simulink model "Yaw_Gearbox_Testrig"  (Simulink 7.9)
settings: Solver=ode23t  StartTime=0.0  StopTime=300  RelTol=1e-3
undefined symbols (not defined in the file): radps2rpm
libraries: fl_lib x9, nesl_utility x3, simulink x1, Yaw_Gearbox_Lib x1
Description:
  | Copyright 2011 MathWorks, Inc.
settings Model: Creator=smiller  LastModifiedBy=smiller
settings DebuggingCC: SolverPrmCheckMsg=none  FcnCallInpInsideContextMsg=Use local settings  StrictBusMsg=Warning
settings GRTTargetCC: CombineOutputUpdateFcns=off  GRTInterface=on

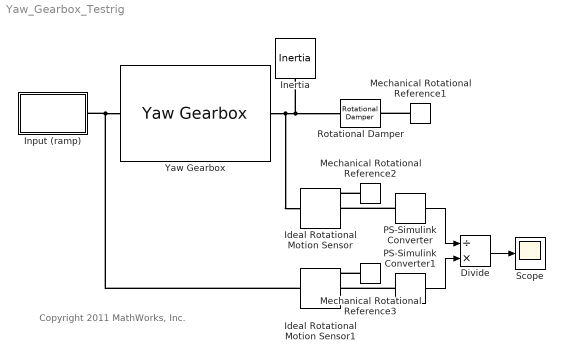
== system Yaw_Gearbox_Testrig ==
  note: Copyright 2011 MathWorks, Inc.
  Divide : Product  Inputs=/*
  Ideal Rotational Motion Sensor : fl_lib/Mechanical/Mechanical Sensors/Ideal Rotational Motion Sensor  offset=0 rad  w_Log=off  t_Log=off  phi_Log=off  LocalVarNames=|w|t|phi  LocalVarDescs=|w|t|phi  LocalVarLogging=[0 0 0]
  Ideal Rotational Motion Sensor1 : fl_lib/Mechanical/Mechanical Sensors/Ideal Rotational Motion Sensor  offset=0 rad  w_Log=off  t_Log=off  phi_Log=off  LocalVarNames=|w|t|phi  LocalVarDescs=|w|t|phi  LocalVarLogging=[0 0 0]
  Inertia : fl_lib/Mechanical/Rotational Elements/Inertia  inertia=1e5 kg*m^2  initial_velocity=0 rad/s  t_Log=off  LocalVarNames=|t  LocalVarDescs=|t  LocalVarLogging=0
  Input (ramp) : Subsystem  mask{start_speed=0, final_speed=14.3004, start_time=3, stop_time=10}
      mask prompts: start_speed "Start speed (rpm)"; final_speed "Final speed (rpm)"; start_time "Ramp start time"; stop_time "Ramp stop time"
  Mechanical Rotational Reference1 : fl_lib/Mechanical/Rotational Elements/Mechanical Rotational Reference  t_Log=off  LocalVarNames=|t  LocalVarDescs=|t  LocalVarLogging=0
  Mechanical Rotational Reference2 : fl_lib/Mechanical/Rotational Elements/Mechanical Rotational Reference  t_Log=off  LocalVarNames=|t  LocalVarDescs=|t  LocalVarLogging=0
  Mechanical Rotational Reference3 : fl_lib/Mechanical/Rotational Elements/Mechanical Rotational Reference  t_Log=off  LocalVarNames=|t  LocalVarDescs=|t  LocalVarLogging=0
  PS-Simulink Converter : nesl_utility/PS-Simulink Converter  PhysicalDomain=network_engine_domain  LeftPortType=input  RightPortType=output  SubClassName=ps_output  Unit=1  AffineConversion=off
  PS-Simulink Converter1 : nesl_utility/PS-Simulink Converter  PhysicalDomain=network_engine_domain  LeftPortType=input  RightPortType=output  SubClassName=ps_output  Unit=1  AffineConversion=off
  Rotational Damper : fl_lib/Mechanical/Rotational Elements/Rotational Damper  D=1000 N*m/(rad/s)  t_Log=off  w_Log=off  LocalVarNames=|t|w  LocalVarDescs=|t|w  LocalVarLogging=[0 0]
  Scope : Scope
      settings: TimeRange=300  YMin=224.0322722113519  YMax=310.1985307541795
  Yaw Gearbox : Yaw_Gearbox_Lib/Yaw Gearbox  SystemSampleTime=-1
  wires:
  Divide/1 -> Scope/1
  PS-Simulink Converter/1 -> Divide/1
  PS-Simulink Converter1/1 -> Divide/2
  connections:
  Yaw Gearbox/LConn1 -- Input (ramp)/LConn1 -- Ideal Rotational Motion Sensor1/LConn1
  Yaw Gearbox/RConn1 -- Inertia/LConn1 -- Rotational Damper/LConn1 -- Ideal Rotational Motion Sensor/LConn1
  Mechanical Rotational Reference1/LConn1 -- Rotational Damper/RConn1
  Mechanical Rotational Reference2/LConn1 -- Ideal Rotational Motion Sensor/RConn1
  Mechanical Rotational Reference3/LConn1 -- Ideal Rotational Motion Sensor1/RConn1
  PS-Simulink Converter/LConn1 -- Ideal Rotational Motion Sensor/RConn2
  PS-Simulink Converter1/LConn1 -- Ideal Rotational Motion Sensor1/RConn2

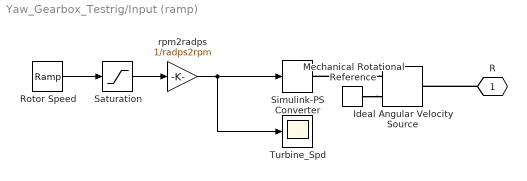
== system Yaw_Gearbox_Testrig/Input (ramp) ==
  Ideal Angular Velocity Source : fl_lib/Mechanical/Mechanical Sources/Ideal Angular Velocity Source  w_Log=off  t_Log=off  LocalVarNames=|w|t  LocalVarDescs=|w|t  LocalVarLogging=[0 0]
  Mechanical Rotational Reference : fl_lib/Mechanical/Rotational Elements/Mechanical Rotational Reference  t_Log=off  LocalVarNames=|t  LocalVarDescs=|t  LocalVarLogging=0
  Rotor Speed : simulink/Sources/Ramp  slope=(final_speed-start_speed)/(stop_time-start_time)  start=start_time  X0=start_speed
  Saturation : Saturate  UpperLimit=final_speed  LowerLimit=0
  Simulink-PS Converter : nesl_utility/Simulink-PS Converter  PhysicalDomain=network_engine_domain  LeftPortType=input  RightPortType=output  SubClassName=ps_input  Unit=1  AffineConversion=off  InputFilterTimeConstant=.001  UdotUserProvided=1  SimscapeFilterOrder=1  InputFiltering=on
  Turbine_Spd : Scope
      settings: YMin=0  YMax=1.5
  rpm2radps : Gain  Gain=1/radps2rpm
  R : PMIOPort  Tag=PMCPort  Port=1  Side=Left
  wires:
  Rotor Speed/1 -> Saturation/1
  Saturation/1 -> rpm2radps/1
  rpm2radps/1 -> Turbine_Spd/1, Simulink-PS Converter/1
  connections:
  R/RConn1 -- Ideal Angular Velocity Source/LConn1
  Ideal Angular Velocity Source/RConn1 -- Simulink-PS Converter/RConn1
  Mechanical Rotational Reference/LConn1 -- Ideal Angular Velocity Source/RConn2
